simulink model "ex_5_sim"  (R2023b)
settings: Solver=FixedStepAuto  StartTime=0.0  StopTime=10  FixedStep=0.01  RelTol=1e-3
values from neighbouring files (symbols this model uses):
  K_1 = 7    [ex_5.m]
  K_2 = 7    [ex_5.m]
  K_3 = 0.1    [ex_5.m]
  q_i = [1 1 pi/4]'    [ex_5.m]
  T_s = 0.01    [ex_5.m]
libraries: robotmobilelib x1
settings Model: Creator=savio  LastModifiedBy=savio

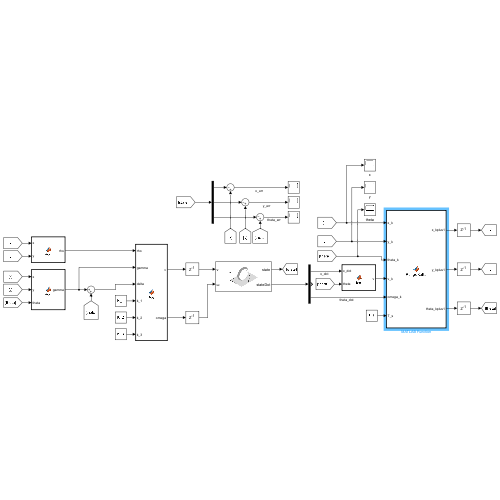
[thumbnail: Simulink's stored preview of the top-level diagram]
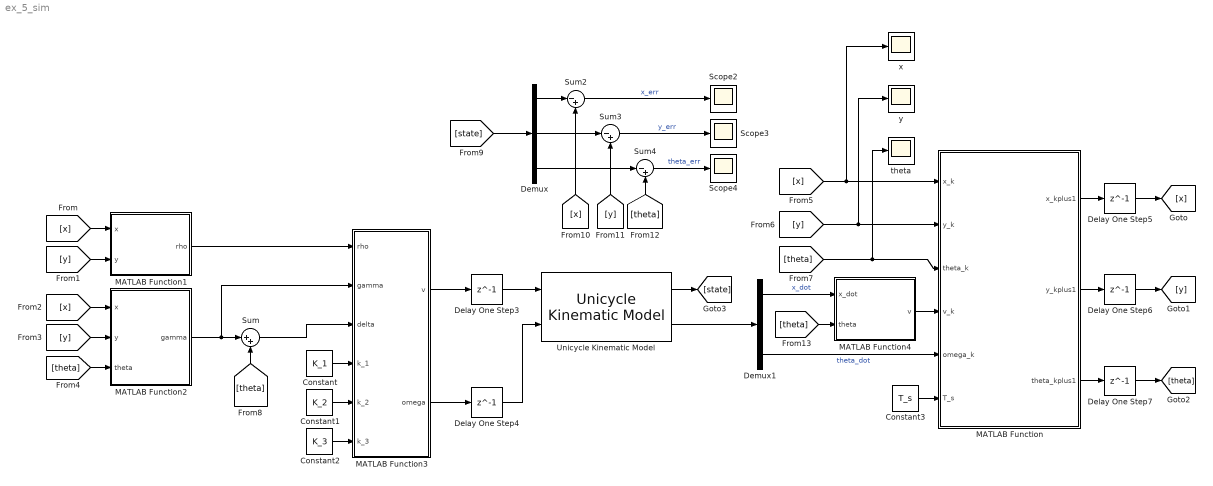
== system ex_5_sim ==
  Constant : Constant  Value=K_1
  Constant1 : Constant  Value=K_2
  Constant2 : Constant  Value=K_3
  Constant3 : Constant  Value=T_s
  Delay One Step3 : Delay  DelayLength=1  InitialCondition=0
  Delay One Step4 : Delay  DelayLength=1  InitialCondition=0
  Delay One Step5 : Delay  DelayLength=1  InitialCondition=q_i(1)
  Delay One Step6 : Delay  DelayLength=1  InitialCondition=q_i(2)
  Delay One Step7 : Delay  DelayLength=1  InitialCondition=q_i(3)
  Demux : Demux  Outputs=3
  Demux1 : Demux  Outputs=3
  MATLAB Function : MATLAB Function  TreatAsAtomicUnit=on
  MATLAB Function1 : MATLAB Function  TreatAsAtomicUnit=on
  MATLAB Function2 : MATLAB Function  TreatAsAtomicUnit=on
  MATLAB Function3 : MATLAB Function  TreatAsAtomicUnit=on
  MATLAB Function4 : MATLAB Function  TreatAsAtomicUnit=on
  Scope2 : Scope
  Scope3 : Scope
  Scope4 : Scope
  Sum : Sum  Inputs=|++
  Sum2 : Sum  Inputs=|-+
  Sum3 : Sum  Inputs=|-+
  Sum4 : Sum  Inputs=|-+
  Unicycle Kinematic Model : robotmobilelib/Unicycle Kinematic Model  VehicleInputs=Vehicle Speed & Heading Angular Velocity  WheelRadius=0.1  WheelSpeedRange=[-Inf Inf]  InitialState=q_i  SimulateUsing=Interpreted execution
  theta : Scope
  x : Scope
  y : Scope
  wires:
  MATLAB Function1/1(rho) -> MATLAB Function3/1(rho)
  MATLAB Function2/1(gamma) -> MATLAB Function3/2(gamma), Sum/1
  Constant/1 -> MATLAB Function3/4(k_1)
  Constant1/1 -> MATLAB Function3/5(k_2)
  Constant2/1 -> MATLAB Function3/6(k_3)
  MATLAB Function3/1(v) -> Delay One Step3/1
  MATLAB Function3/2(omega) -> Delay One Step4/1
  [x] -> MATLAB Function1/1(x)
  [y] -> MATLAB Function1/2(y)
  [x] -> MATLAB Function2/1(x)
  [y] -> MATLAB Function2/2(y)
  [theta] -> MATLAB Function2/3(theta)
  Unicycle Kinematic Model/2 -> Demux1/1
  Demux1/3 -> MATLAB Function/5(omega_k)  "theta_dot"
  Constant3/1 -> MATLAB Function/6(T_s)
  Delay One Step3/1 -> Unicycle Kinematic Model/1
  Delay One Step4/1 -> Unicycle Kinematic Model/2
  Sum/1 -> MATLAB Function3/3(delta)
  Demux1/1 -> MATLAB Function4/1(x_dot)  "x_dot"
  MATLAB Function4/1(v) -> MATLAB Function/4(v_k)
  MATLAB Function/1(x_kplus1) -> Delay One Step5/1
  MATLAB Function/2(y_kplus1) -> Delay One Step6/1
  MATLAB Function/3(theta_kplus1) -> Delay One Step7/1
  [x] -> MATLAB Function/1(x_k), x/1
  [y] -> MATLAB Function/2(y_k), y/1
  [theta] -> MATLAB Function/3(theta_k), theta/1
  Unicycle Kinematic Model/1 -> [state]
  [state] -> Demux/1
  [x] -> Sum2/2
  [y] -> Sum3/2
  [theta] -> Sum4/2
  Demux/1 -> Sum2/1
  Demux/2 -> Sum3/1
  Demux/3 -> Sum4/1
  Sum4/1 -> Scope4/1  "theta_err"
  Sum3/1 -> Scope3/1  "y_err"
  Sum2/1 -> Scope2/1  "x_err"
  [theta] -> Sum/2
  Delay One Step5/1 -> [x]
  Delay One Step6/1 -> [y]
  Delay One Step7/1 -> [theta]
  [theta] -> MATLAB Function4/2(theta)

== matlab function ex_5_sim/MATLAB Function1 ==
  data: x input; rho output; y input
function rho = fcn(x, y)
rho = sqrt(x^2+y^2);

== matlab function ex_5_sim/MATLAB Function ==
  data: x_k input; x_kplus1 output; y_k input; theta_k input; v_k input; omega_k input; T_s input; y_kplus1 output; theta_kplus1 output
function [x_kplus1, y_kplus1, theta_kplus1] = RungeKutta(x_k, y_k, theta_k, v_k, omega_k, T_s)

x_kplus1 = x_k + v_k*T_s*cos(theta_k+omega_k*T_s/2);
y_kplus1 = y_k + v_k*T_s*sin(theta_k+omega_k*T_s/2);
theta_kplus1 = theta_k + omega_k*T_s;

== matlab function ex_5_sim/MATLAB Function2 ==
  data: x input; gamma output; y input; theta input
function gamma = fcn(x, y, theta)
gamma = atan2(y,x) - theta + pi;

== matlab function ex_5_sim/MATLAB Function3 ==
  data: rho input; v output; gamma input; delta input; k_1 input; k_2 input; k_3 input; omega output
function [v, omega] = fcn(rho, gamma, delta, k_1, k_2, k_3)

v = k_1*rho*cos(gamma);
omega = k_2*gamma + k_1*sin(gamma)*cos(gamma)*(1 + k_3*delta/gamma);

== matlab function ex_5_sim/MATLAB Function4 ==
  data: x_dot input; v output; theta input
function v = fcn(x_dot, theta)

v = x_dot/cos(theta)
